simulink model "CryoDetMultiChan_CMB"  (R2016b)
settings: Solver=ode45  StartTime=0.0  StopTime=400e-6  MaxStep=Tclk/4  RelTol=1e-3
values from neighbouring files (symbols this model uses):
  ds_axi = 16    [setupCryoFPGA_CMB.m]
  Fclk = Fadc    (= 307200000)    [setupCryoFPGA_CMB.m]
  lpf = tf(num,den)    [setupCryoFPGA_CMB.m]
  Tclk = 1/Fclk    (= 3.25520833333e-09)    [setupCryoFPGA_CMB.m]
  Ts = 1/Fs    (= 3.25520833333e-09)    [setupADCtoDACloopback.m]    (also in setupCryoFPGA_CMB.m)
undefined symbols (not defined in the file or in its folder): AXI4, i, Lite, xlipgetpartsetting
libraries: xbsIndex_r4 x2215, hdlsllib x6, simulink x3, CryoDetLib x2
(part 5 of 16)

== system CryoDetMultiChan_CMB/DspCore/FTA_Ch0/SixteenLineUDC 0 ==
  note: REF I & Q are in original (unswapped)
      | configuration
  note: SixteenLineUDC(n)
      |
      | Implelents the Up *and* Down Conversion for each Resonator Line/Channel
      | One Block implements one U/D converter pair
      | The counter use used to syncronize the internal CIC filter reset operation to allow the data to be interleaved
      | The MUX16x4 block does the actual time-domain interleaving operation
      | The DC Decimate block does a further decimate and filtering operation on the ADC and Reference signals before sending them downstream for furhter processing
      | The DAC SUM block individually sums the I & Q components of the upconverted signals (4 individual sum streams from the DAC & DAC + phi signals) before they are forwarded downstream.
  ADC_I_in : Inport
  ADC_Q_in : Inport  Port=2
  REF_I_in1 : Inport  Port=3
  REF_Q_in1 : Inport  Port=4
  BDC scope : Scope  NumInputPorts=2
  Constant : xbsIndex_r4/Constant  const=0  gui_display_data_type=Fixed-point  arith_type=Unsigned  n_bits=5  bin_pt=0  preci_type=Single  exp_width=8  frac_width=24  explicit_period=off  period=1  equ=P=C  opselect=C  inp2=PCIN>>17  opr=+  inp1=P  carry=CIN  dbl_ovrd=off  block_type=constant
  Constant1 : xbsIndex_r4/Constant  const=1  gui_display_data_type=Fixed-point  arith_type=Unsigned  n_bits=5  bin_pt=0  preci_type=Single  exp_width=8  frac_width=24  explicit_period=off  period=1  equ=P=C  opselect=C  inp2=PCIN>>17  opr=+  inp1=P  carry=CIN  dbl_ovrd=off  block_type=constant
  Constant10 : xbsIndex_r4/Constant  const=10  gui_display_data_type=Fixed-point  arith_type=Unsigned  n_bits=5  bin_pt=0  preci_type=Single  exp_width=8  frac_width=24  explicit_period=off  period=1  equ=P=C  opselect=C  inp2=PCIN>>17  opr=+  inp1=P  carry=CIN  dbl_ovrd=off  block_type=constant
  Constant11 : xbsIndex_r4/Constant  const=11  gui_display_data_type=Fixed-point  arith_type=Unsigned  n_bits=5  bin_pt=0  preci_type=Single  exp_width=8  frac_width=24  explicit_period=off  period=1  equ=P=C  opselect=C  inp2=PCIN>>17  opr=+  inp1=P  carry=CIN  dbl_ovrd=off  block_type=constant
  Constant12 : xbsIndex_r4/Constant  const=12  gui_display_data_type=Fixed-point  arith_type=Unsigned  n_bits=5  bin_pt=0  preci_type=Single  exp_width=8  frac_width=24  explicit_period=off  period=1  equ=P=C  opselect=C  inp2=PCIN>>17  opr=+  inp1=P  carry=CIN  dbl_ovrd=off  block_type=constant
  Constant13 : xbsIndex_r4/Constant  const=13  gui_display_data_type=Fixed-point  arith_type=Unsigned  n_bits=5  bin_pt=0  preci_type=Single  exp_width=8  frac_width=24  explicit_period=off  period=1  equ=P=C  opselect=C  inp2=PCIN>>17  opr=+  inp1=P  carry=CIN  dbl_ovrd=off  block_type=constant
  Constant14 : xbsIndex_r4/Constant  const=14  gui_display_data_type=Fixed-point  arith_type=Unsigned  n_bits=5  bin_pt=0  preci_type=Single  exp_width=8  frac_width=24  explicit_period=off  period=1  equ=P=C  opselect=C  inp2=PCIN>>17  opr=+  inp1=P  carry=CIN  dbl_ovrd=off  block_type=constant
  Constant15 : xbsIndex_r4/Constant  const=15  gui_display_data_type=Fixed-point  arith_type=Unsigned  n_bits=5  bin_pt=0  preci_type=Single  exp_width=8  frac_width=24  explicit_period=off  period=1  equ=P=C  opselect=C  inp2=PCIN>>17  opr=+  inp1=P  carry=CIN  dbl_ovrd=off  block_type=constant
  Constant2 : xbsIndex_r4/Constant  const=2  gui_display_data_type=Fixed-point  arith_type=Unsigned  n_bits=5  bin_pt=0  preci_type=Single  exp_width=8  frac_width=24  explicit_period=off  period=1  equ=P=C  opselect=C  inp2=PCIN>>17  opr=+  inp1=P  carry=CIN  dbl_ovrd=off  block_type=constant
  Constant20 : xbsIndex_r4/Constant  const=31  gui_display_data_type=Fixed-point  arith_type=Unsigned  n_bits=5  bin_pt=0  preci_type=Single  exp_width=8  frac_width=24  explicit_period=off  period=1  equ=P=C  opselect=C  inp2=PCIN>>17  opr=+  inp1=P  carry=CIN  dbl_ovrd=off  block_type=constant
  Constant3 : xbsIndex_r4/Constant  const=3  gui_display_data_type=Fixed-point  arith_type=Unsigned  n_bits=5  bin_pt=0  preci_type=Single  exp_width=8  frac_width=24  explicit_period=off  period=1  equ=P=C  opselect=C  inp2=PCIN>>17  opr=+  inp1=P  carry=CIN  dbl_ovrd=off  block_type=constant
  Constant4 : xbsIndex_r4/Constant  const=4  gui_display_data_type=Fixed-point  arith_type=Unsigned  n_bits=5  bin_pt=0  preci_type=Single  exp_width=8  frac_width=24  explicit_period=off  period=1  equ=P=C  opselect=C  inp2=PCIN>>17  opr=+  inp1=P  carry=CIN  dbl_ovrd=off  block_type=constant
  Constant5 : xbsIndex_r4/Constant  const=5  gui_display_data_type=Fixed-point  arith_type=Unsigned  n_bits=5  bin_pt=0  preci_type=Single  exp_width=8  frac_width=24  explicit_period=off  period=1  equ=P=C  opselect=C  inp2=PCIN>>17  opr=+  inp1=P  carry=CIN  dbl_ovrd=off  block_type=constant
  Constant6 : xbsIndex_r4/Constant  const=6  gui_display_data_type=Fixed-point  arith_type=Unsigned  n_bits=5  bin_pt=0  preci_type=Single  exp_width=8  frac_width=24  explicit_period=off  period=1  equ=P=C  opselect=C  inp2=PCIN>>17  opr=+  inp1=P  carry=CIN  dbl_ovrd=off  block_type=constant
  Constant7 : xbsIndex_r4/Constant  const=7  gui_display_data_type=Fixed-point  arith_type=Unsigned  n_bits=5  bin_pt=0  preci_type=Single  exp_width=8  frac_width=24  explicit_period=off  period=1  equ=P=C  opselect=C  inp2=PCIN>>17  opr=+  inp1=P  carry=CIN  dbl_ovrd=off  block_type=constant
  Constant8 : xbsIndex_r4/Constant  const=8  gui_display_data_type=Fixed-point  arith_type=Unsigned  n_bits=5  bin_pt=0  preci_type=Single  exp_width=8  frac_width=24  explicit_period=off  period=1  equ=P=C  opselect=C  inp2=PCIN>>17  opr=+  inp1=P  carry=CIN  dbl_ovrd=off  block_type=constant
  Constant9 : xbsIndex_r4/Constant  const=9  gui_display_data_type=Fixed-point  arith_type=Unsigned  n_bits=5  bin_pt=0  preci_type=Single  exp_width=8  frac_width=24  explicit_period=off  period=1  equ=P=C  opselect=C  inp2=PCIN>>17  opr=+  inp1=P  carry=CIN  dbl_ovrd=off  block_type=constant
  Counter : xbsIndex_r4/Counter  cnt_type=Count Limited  cnt_to=31  operation=Up  start_count=0  cnt_by_val=1  arith_type=Unsigned  n_bits=5  bin_pt=0  load_pin=off  rst=on  en=on  explicit_period=off  period=Tclk  use_behavioral_HDL=off  implementation=Fabric  dbl_ovrd=off  block_type=counter
  DAC Sum1 : Subsystem
  DC_decimate : Subsystem
  Delay : xbsIndex_r4/Delay  rst=off  infoeditControl=Selection of Reset will increase slice count due to use of real FFs and instead of SRLs  en=off  latency=6  reg_retiming=off  dbl_ovrd=off  block_type=delay
  Demux : Demux  Outputs=2
  Demux1 : Demux  Outputs=2
  Gateway Out{1,7..10,23} (6 alike) : xbsIndex_r4/Gateway Out  inherit_from_input=off  hdl_port=off  rows=1  columns=1  UseAsDAC=off  DACChannel='1'  interface=None  automatic_assignment=on  address_offset=hex2dec('00')  intf_name=''  intf_description=''  timing_constraint=None  locs_specified=off  LOCs={}  io_standard={}  block_type=gatewayout
  Mux{,1,6..7} (4 alike) : Mux  Inputs=2
  Mux16X4 : Subsystem
  Relational : xbsIndex_r4/Relational  mode=a!=b  op_type=Bool  en=off  latency=0  dbl_ovrd=off  block_type=relational
  debug Scope : Subsystem
  oneLineUpDown0 : Subsystem
  oneLineUpDown1 : Subsystem
  oneLineUpDown10 : Subsystem
  oneLineUpDown11 : Subsystem
  oneLineUpDown12 : Subsystem
  oneLineUpDown13 : Subsystem
  oneLineUpDown14 : Subsystem
  oneLineUpDown15 : Subsystem
  oneLineUpDown2 : Subsystem
  oneLineUpDown3 : Subsystem
  oneLineUpDown4 : Subsystem
  oneLineUpDown5 : Subsystem
  oneLineUpDown6 : Subsystem
  oneLineUpDown7 : Subsystem
  oneLineUpDown8 : Subsystem
  oneLineUpDown9 : Subsystem
  synch scope : Scope  NumInputPorts=2
  toDAC : Outport
  demodulated : Outport  Port=2
  wires:
  [fpgaReset] -> Counter/1, Delay/1
  Gateway Out10/1 -> Mux7/2
  Gateway Out9/1 -> Mux7/1
  Gateway Out8/1 -> Mux6/2
  Gateway Out7/1 -> Mux6/1
  Mux6/1 -> BDC scope/1
  Mux7/1 -> BDC scope/2
  Demux/1 -> Gateway Out7/1
  Demux1/2 -> Gateway Out10/1
  Demux1/1 -> Gateway Out9/1
  Demux/2 -> Gateway Out8/1
  Delay/1 -> Mux16X4/1(synch)
  Constant/1 -> oneLineUpDown0/2(addrIn)
  Counter/1 -> Gateway Out23/1, oneLineUpDown1/3(synchIn), oneLineUpDown2/3(synchIn), oneLineUpDown3/3(synchIn), oneLineUpDown4/3(synchIn), oneLineUpDown5/3(synchIn), oneLineUpDown6/3(synchIn), oneLineUpDown7/3(synchIn), oneLineUpDown8/3(synchIn), oneLineUpDown9/3(synchIn), oneLineUpDown10/3(synchIn), oneLineUpDown11/3(synchIn), oneLineUpDown12/3(synchIn), oneLineUpDown13/3(synchIn), oneLineUpDown15/3(synchIn), oneLineUpDown14/3(synchIn), oneLineUpDown0/3(synchIn), Relational/2
  Gateway Out23/1 -> synch scope/1
  Gateway Out1/1 -> synch scope/2
  Relational/1 -> Gateway Out1/1, Counter/2
  Constant20/1 -> Relational/1
  oneLineUpDown0/1(DC_Out) -> debug Scope/1(demod), Mux16X4/2(line0)  "DC_out_line0"
  oneLineUpDown1/1(DC_Out) -> Mux16X4/3(line1)  "DC_out_line1"
  oneLineUpDown2/1(DC_Out) -> Mux16X4/4(line2)  "DC_out_line2"
  oneLineUpDown3/1(DC_Out) -> Mux16X4/5(line3)  "DC_out_line3"
  oneLineUpDown4/1(DC_Out) -> Mux16X4/6(line4)  "DC_out_line4"
  oneLineUpDown5/1(DC_Out) -> Mux16X4/7(line5)  "DC_out_line5"
  oneLineUpDown6/1(DC_Out) -> Mux16X4/8(line6)  "DC_out_line6"
  oneLineUpDown7/1(DC_Out) -> Mux16X4/9(line7)  "DC_out_line7"
  oneLineUpDown8/1(DC_Out) -> Mux16X4/10(line8)  "DC_out_line8"
  oneLineUpDown9/1(DC_Out) -> Mux16X4/11(line9)  "DC_out_line9"
  oneLineUpDown10/1(DC_Out) -> Mux16X4/12(line10)  "DC_out_line10"
  oneLineUpDown11/1(DC_Out) -> Mux16X4/13(line11)  "DC_out_line11"
  oneLineUpDown12/1(DC_Out) -> Mux16X4/14(line12)  "DC_out_line12"
  oneLineUpDown13/1(DC_Out) -> Mux16X4/15(line13)  "DC_out_line13"
  oneLineUpDown14/1(DC_Out) -> Mux16X4/16(line14)  "DC_out_line14"
  oneLineUpDown15/1(DC_Out) -> Mux16X4/17(line15)  "DC_out_line15"
  oneLineUpDown15/2(UC_out) -> DAC Sum1/1(In1)  "UC_out_line15"
  oneLineUpDown14/2(UC_out) -> DAC Sum1/2(In2)  "UC_out_line14"
  oneLineUpDown13/2(UC_out) -> DAC Sum1/3(In3)  "UC_out_line13"
  oneLineUpDown12/2(UC_out) -> DAC Sum1/4(In4)  "UC_out_line12"
  oneLineUpDown11/2(UC_out) -> DAC Sum1/5(In5)  "UC_out_line11"
  oneLineUpDown10/2(UC_out) -> DAC Sum1/6(In6)  "UC_out_line10"
  oneLineUpDown9/2(UC_out) -> DAC Sum1/7(In7)  "UC_out_line9"
  oneLineUpDown8/2(UC_out) -> DAC Sum1/8(In8)  "UC_out_line8"
  oneLineUpDown7/2(UC_out) -> DAC Sum1/9(In9)  "UC_out_line7"
  oneLineUpDown6/2(UC_out) -> DAC Sum1/10(In10)  "UC_out_line6"
  oneLineUpDown5/2(UC_out) -> DAC Sum1/11(In11)  "UC_out_line5"
  oneLineUpDown4/2(UC_out) -> DAC Sum1/12(In12)  "UC_out_line4"
  oneLineUpDown3/2(UC_out) -> DAC Sum1/13(In13)  "UC_out_line3"
  oneLineUpDown2/2(UC_out) -> DAC Sum1/14(In14)  "UC_out_line2"
  oneLineUpDown1/2(UC_out) -> DAC Sum1/15(In15)  "UC_out_line1"
  oneLineUpDown0/3(UC_out) -> DAC Sum1/16(In16)  "UC_out_line0"
  Constant1/1 -> oneLineUpDown1/2(addrIn)
  Constant2/1 -> oneLineUpDown2/2(addrIn)
  Constant3/1 -> oneLineUpDown3/2(addrIn)
  Constant4/1 -> oneLineUpDown4/2(addrIn)
  Constant5/1 -> oneLineUpDown5/2(addrIn)
  Constant6/1 -> oneLineUpDown6/2(addrIn)
  Constant7/1 -> oneLineUpDown7/2(addrIn)
  Constant8/1 -> oneLineUpDown8/2(addrIn)
  Constant9/1 -> oneLineUpDown9/2(addrIn)
  Constant10/1 -> oneLineUpDown10/2(addrIn)
  Constant11/1 -> oneLineUpDown11/2(addrIn)
  Constant12/1 -> oneLineUpDown12/2(addrIn)
  Constant13/1 -> oneLineUpDown13/2(addrIn)
  Constant14/1 -> oneLineUpDown14/2(addrIn)
  Constant15/1 -> oneLineUpDown15/2(addrIn)
  ADC_Q_in/1 -> Mux/1
  ADC_I_in/1 -> Mux/2
  REF_I_in1/1 -> Mux1/2
  REF_Q_in1/1 -> Mux1/1
  Mux/1 -> oneLineUpDown1/1(ADC_IQ_in), oneLineUpDown2/1(ADC_IQ_in), Demux/1, oneLineUpDown3/1(ADC_IQ_in), oneLineUpDown4/1(ADC_IQ_in), oneLineUpDown5/1(ADC_IQ_in), oneLineUpDown6/1(ADC_IQ_in), oneLineUpDown7/1(ADC_IQ_in), oneLineUpDown8/1(ADC_IQ_in), oneLineUpDown9/1(ADC_IQ_in), oneLineUpDown10/1(ADC_IQ_in), oneLineUpDown11/1(ADC_IQ_in), oneLineUpDown12/1(ADC_IQ_in), oneLineUpDown13/1(ADC_IQ_in), oneLineUpDown15/1(ADC_IQ_in), oneLineUpDown14/1(ADC_IQ_in), oneLineUpDown0/1(ADC_IQ_in)
  Mux1/1 -> oneLineUpDown0/4(REF_IQ_in1), oneLineUpDown1/4(REF_IQ_in1), oneLineUpDown2/4(REF_IQ_in1), oneLineUpDown3/4(REF_IQ_in1), oneLineUpDown4/4(REF_IQ_in1), Demux1/1, oneLineUpDown5/4(REF_IQ_in1), oneLineUpDown6/4(REF_IQ_in1), oneLineUpDown7/4(REF_IQ_in1), oneLineUpDown8/4(REF_IQ_in1), oneLineUpDown9/4(REF_IQ_in1), oneLineUpDown10/4(REF_IQ_in1), oneLineUpDown11/4(REF_IQ_in1), oneLineUpDown12/4(REF_IQ_in1), oneLineUpDown13/4(REF_IQ_in1), oneLineUpDown15/4(REF_IQ_in1), oneLineUpDown14/4(REF_IQ_in1)
  DAC Sum1/1(Out1) -> toDAC/1
  Mux16X4/1(Out1) -> DC_decimate/1(In1)
  DC_decimate/1(dec_sig_ref) -> demodulated/1
  oneLineUpDown0/2(Freq) -> debug Scope/2(freq)

== system CryoDetMultiChan_CMB/DspCore/FTA_Ch0/dF ==
  note: NOTE <11-08-2017 JED>: Connected RE{} output to dFBus now instead of IM{} as was originally
  note: Latency =11
  note: Delay4 + eta mux + cast/covnert total latency = 19
      |
      | Note: this path should match above (multiply) path
  note: Channel
  note: sig0
  note: conj(Ref0)
  note: Match latencies
  note: dF
  note: Ref
  note: Sig
  note: Frequency error dF = Re(eta'*Ref'*Sig)
      | where eta' is like a phase and amplitude calibration including the phase determined by the 2 sidebands and amplitude determined by the reference central line and bandwidth
      |
      | get channel ID
      | fetch eta'
      | calc dF
      | dF now Re{} w/o sidebands <JED: 11-08-2017>
  note: Tvalid
  note: eta mux has latency of 4
  note: Latency =11
  In1 : Inport
  BW : Display
  BW in MHz : Display
  Bus Creator : BusCreator  Inputs=3
  Bus Selector : BusSelector  OutputSignals=chanAndTvalid,decSigandRef
  Bus Selector4 : BusSelector  OutputSignals=Q_Eta,I_Eta
  CMult : xbsIndex_r4/CMult  const=-1  gui_display_data_type=Floating-point  const_n_bits=24  const_bin_pt=22  float_type=Single  exp_bits=8  fraction_bits=24  en=off  latency=3  precision=Full  arith_type="Signed  (2's comp)"  n_bits=24  bin_pt=22  quantization=Truncate  overflow=Wrap  use_behavioral_HDL=on  mem_type=Distributed RAM  pipeline=off  dbl_ovrd=off  block_type=cmult
  Constant : xbsIndex_r4/Constant  const=0  gui_display_data_type=Fixed-point  arith_type=Unsigned  n_bits=4  bin_pt=0  preci_type=Single  exp_width=8  frac_width=24  explicit_period=off  period=1  equ=P=C  opselect=C  inp2=PCIN>>17  opr=+  inp1=P  carry=CIN  dbl_ovrd=off  block_type=constant
  Constant1 : xbsIndex_r4/Constant  const=0  gui_display_data_type=Fixed-point  arith_type=Unsigned  n_bits=4  bin_pt=0  preci_type=Single  exp_width=8  frac_width=24  explicit_period=off  period=1  equ=P=C  opselect=C  inp2=PCIN>>17  opr=+  inp1=P  carry=CIN  dbl_ovrd=off  block_type=constant
  Convert{,1..3,6..7} (6 alike) : xbsIndex_r4/Convert  gui_display_data_type=Floating-point  arith_type=Floating-point  n_bits=16  bin_pt=14  float_type=Single  exp_bits=8  fraction_bits=24  quantization=Truncate  overflow=Wrap  en=off  latency=5  pipeline=off  dbl_ovrd=off  block_type=convert
  Convert10 : xbsIndex_r4/Convert  gui_display_data_type=Fixed-point  arith_type="Signed  (2's comp)"  n_bits=32  bin_pt=30  float_type=Single  exp_bits=8  fraction_bits=24  quantization="Round  (unbiased: +/- Inf)"  overflow=Saturate  en=off  latency=2  pipeline=on  dbl_ovrd=off  block_type=convert
  Convert{8..9,11..13} (5 alike) : xbsIndex_r4/Convert  gui_display_data_type=Fixed-point  arith_type="Signed  (2's comp)"  n_bits=32  bin_pt=30  float_type=Single  exp_bits=8  fraction_bits=24  quantization="Round  (unbiased: +/- Inf)"  overflow=Saturate  en=off  latency=1  pipeline=off  dbl_ovrd=off  block_type=convert
  Convert4 : xbsIndex_r4/Convert  gui_display_data_type=Fixed-point  arith_type="Signed  (2's comp)"  n_bits=32  bin_pt=30  float_type=Single  exp_bits=8  fraction_bits=24  quantization="Round  (unbiased: +/- Inf)"  overflow=Saturate  en=off  latency=2  pipeline=on  dbl_ovrd=off  block_type=convert
  Convert5 : xbsIndex_r4/Convert  gui_display_data_type=Floating-point  arith_type=Floating-point  n_bits=16  bin_pt=14  float_type=Single  exp_bits=8  fraction_bits=24  quantization=Truncate  overflow=Wrap  en=off  latency=4  pipeline=on  dbl_ovrd=off  block_type=convert
  CplxProd : Subsystem
  CplxProd1 : Subsystem
  Delay : xbsIndex_r4/Delay  rst=off  infoeditControl=Selection of Reset will increase slice count due to use of real FFs and instead of SRLs  en=off  latency=3  reg_retiming=on  dbl_ovrd=off  block_type=delay
  Delay1 : xbsIndex_r4/Delay  rst=off  infoeditControl=Selection of Reset will increase slice count due to use of real FFs and instead of SRLs  en=off  latency=3  reg_retiming=on  dbl_ovrd=off  block_type=delay
  Delay2 : xbsIndex_r4/Delay  rst=off  infoeditControl=Selection of Reset will increase slice count due to use of real FFs and instead of SRLs  en=off  latency=3  reg_retiming=on  dbl_ovrd=off  block_type=delay
  Delay3 : xbsIndex_r4/Delay  rst=off  infoeditControl=Selection of Reset will increase slice count due to use of real FFs and instead of SRLs  en=off  latency=36  reg_retiming=on  dbl_ovrd=off  block_type=delay
  Delay4 : xbsIndex_r4/Delay  rst=off  infoeditControl=Selection of Reset will increase slice count due to use of real FFs and instead of SRLs  en=off  latency=10  reg_retiming=on  dbl_ovrd=off  block_type=delay
  Delay5 : xbsIndex_r4/Delay  rst=off  infoeditControl=Selection of Reset will increase slice count due to use of real FFs and instead of SRLs  en=off  latency=8  reg_retiming=on  dbl_ovrd=off  block_type=delay
  Delay6 : xbsIndex_r4/Delay  rst=off  infoeditControl=Selection of Reset will increase slice count due to use of real FFs and instead of SRLs  en=off  latency=6  reg_retiming=on  dbl_ovrd=off  block_type=delay
  Demux{1..4} (4 alike) : Demux  Outputs=2
  Display2 : Display
  Display3 : Display
  Gain : Gain  Gain=307.2
  Gateway Out{1..2,4..10} (9 alike) : xbsIndex_r4/Gateway Out  inherit_from_input=off  hdl_port=off  rows=1  columns=1  UseAsDAC=off  DACChannel='1'  interface=None  automatic_assignment=on  address_offset=hex2dec('00')  intf_name=''  intf_description=''  timing_constraint=None  locs_specified=off  LOCs={}  io_standard={}  block_type=gatewayout
  Gateway Out3 : xbsIndex_r4/Gateway Out  inherit_from_input=on  hdl_port=off  rows=1  columns=1  UseAsDAC=off  DACChannel='1'  interface=None  automatic_assignment=on  address_offset=hex2dec('00')  intf_name=''  intf_description=''  timing_constraint=None  locs_specified=off  LOCs={}  io_standard={}  block_type=gatewayout
  Mult1 : xbsIndex_r4/Mult  precision=Full  arith_type="Signed  (2's comp)"  n_bits=32  bin_pt=30  quantization="Round  (unbiased: +/- Inf)"  overflow=Saturate  en=off  latency=4  use_behavioral_HDL=on  opt=Speed  use_embedded=on  optimum_pipeline=off  pipeline=on  dbl_ovrd=off  use_rpm=on  placement_style=Triangular  block_type=mult
  Mult4 : xbsIndex_r4/Mult  precision=Full  arith_type="Signed  (2's comp)"  n_bits=32  bin_pt=30  quantization="Round  (unbiased: +/- Inf)"  overflow=Saturate  en=off  latency=4  use_behavioral_HDL=on  opt=Speed  use_embedded=on  optimum_pipeline=off  pipeline=on  dbl_ovrd=off  use_rpm=on  placement_style=Triangular  block_type=mult
  Register : xbsIndex_r4/Register  init=0  rst=off  en=on  dbl_ovrd=off  block_type=register
  Register1 : xbsIndex_r4/Register  init=0  rst=off  en=off  dbl_ovrd=off  block_type=register
  Register2 : xbsIndex_r4/Register  init=0  rst=off  en=on  dbl_ovrd=off  block_type=register
  Register8 : xbsIndex_r4/Register  init=0  rst=off  en=off  dbl_ovrd=off  block_type=register
  Relational : xbsIndex_r4/Relational  mode=a=b  op_type=Bool  en=off  latency=0  dbl_ovrd=off  block_type=relational
  Relational1 : xbsIndex_r4/Relational  mode=a=b  op_type=Bool  en=off  latency=0  dbl_ovrd=off  block_type=relational
  dF CplxProd1 scope : Scope  NumInputPorts=8
  dF intermediate : Scope  NumInputPorts=8
  dF output : Scope  NumInputPorts=2
  dF scope1 : Scope  NumInputPorts=3
  eta Mux1 : Subsystem
  Out1 : Outport
  tag scope: REAL_ch0_dF_latched=global, ch0_dF_latched=global, dFbus=global
  wires:
  CMult/1 -> CplxProd/4(Im_B)
  Demux2/1 -> Convert2/1
  Demux2/2 -> Convert3/1
  Delay/1 -> CplxProd/5(Re_B)
  Demux1/2 -> Convert1/1
  Demux1/1 -> Convert/1
  Delay1/1 -> CplxProd/2(Im_A)
  CplxProd1/3(Re_Out) -> Mult1/2, dF CplxProd1 scope/7
  Delay6/1 -> dF intermediate/8, Bus Creator/1  "Dvalid"
  In1/1 -> Bus Selector/1
  Bus Creator/1 -> [dFbus], Out1/1
  Register1/1 -> Convert12/1, Mult1/1, Mult4/1, Gateway Out1/1
  CplxProd1/2(Im_Out) -> Convert11/1, dF CplxProd1 scope/8, Mult4/2
  Demux4/1 -> dF scope1/2, Delay3/1, Delay4/1
  Demux4/2 -> dF scope1/1, Delay5/1
  Bus Selector/1 -> Demux4/1  "<chanAndTvalid>"
  Bus Selector/2 -> dF scope1/3, Demux3/1  "<decSigandRef>"
  Mult4/1 -> Convert13/1, Convert4/1  "freqError"
  Delay3/1 -> Gateway Out6/1, Relational1/1, Relational/1, Gateway Out3/1, Bus Creator/2  "channel"
  Convert3/1 -> Delay/1
  Convert2/1 -> CMult/1
  Convert1/1 -> Delay2/1
  Convert/1 -> Delay1/1
  Delay2/1 -> CplxProd/3(Re_A)
  Delay5/1 -> CplxProd/1(tvalidIn)
  CplxProd/2(Im_Out) -> dF CplxProd1 scope/3, CplxProd1/2(Im_A), Convert8/1
  CplxProd/3(Re_Out) -> dF CplxProd1 scope/2, CplxProd1/3(Re_A), Convert9/1
  Convert6/1 -> dF CplxProd1 scope/5, CplxProd1/4(Im_B)
  Convert7/1 -> dF CplxProd1 scope/4, CplxProd1/5(Re_B)
  CplxProd/1(tvalidOut) -> dF CplxProd1 scope/1, CplxProd1/1(tvalidIn)
  Convert4/1 -> dF intermediate/7, Register/1  "old_freqError"
  Gateway Out4/1 -> [ch0_dF_latched], Display3/1, dF output/2
  Gateway Out3/1 -> dF output/1, Display2/1
  Constant/1 -> Relational/2
  Relational/1 -> Register/2
  Register/1 -> Gateway Out4/1
  [BW] -> Register8/1
  Gateway Out1/1 -> BW/1, Gain/1
  Gain/1 -> BW in MHz/1
  Bus Selector4/1 -> Convert6/1  "<Q_Eta>"
  Bus Selector4/2 -> Convert7/1  "<I_Eta>"
  eta Mux1/1(eta out) -> Bus Selector4/1
  Delay4/1 -> eta Mux1/1(channel)
  Demux3/2 -> Demux2/1
  Demux3/1 -> Demux1/1
  Convert9/1 -> Gateway Out2/1
  Convert8/1 -> Gateway Out5/1
  Convert11/1 -> Gateway Out7/1
  Gateway Out2/1 -> dF intermediate/3
  Gateway Out5/1 -> dF intermediate/2
  Gateway Out6/1 -> dF intermediate/1
  Gateway Out7/1 -> dF intermediate/4
  Convert12/1 -> Gateway Out8/1
  Gateway Out8/1 -> dF intermediate/5
  Convert13/1 -> Gateway Out9/1
  Gateway Out9/1 -> dF intermediate/6
  CplxProd1/1(tvalidOut) -> dF CplxProd1 scope/6, Delay6/1  "Dvalid"
  Register8/1 -> Convert5/1
  Convert5/1 -> Register1/1
  Gateway Out10/1 -> [REAL_ch0_dF_latched]
  Constant1/1 -> Relational1/2
  Relational1/1 -> Register2/2
  Register2/1 -> Gateway Out10/1
  Mult1/1 -> Convert10/1
  Convert10/1 -> Register2/1, Bus Creator/3  "freqError"

== system CryoDetMultiChan_CMB/DspCore/FTA_Ch0/dphi ==
  note: check format of Fbus
  note: scale by 1/2 since phase increment per 1/370 = 1/2 of phase increment per 1/185
  note: dPhi
      | calculate complex phase advance for a single sample of ADC input
      | at the frequency of a single channel and send off on dphiBus
  In1 : Inport
  BitBasher : xbsIndex_r4/BitBasher  bitexpr=a={1'b0, b[23:1]}  display_expr=on  sr_1=a  arith_type1=Unsigned  bin_pt1=24  sr_2=2  arith_type2=Unsigned  bin_pt2=0  sr_3=3  arith_type3=Unsigned  bin_pt3=0  sr_4=4  arith_type4=Unsigned  bin_pt4=0  dbl_ovrd=off  block_type=bitbasher
  Bus Creator : BusCreator  Inputs=3
  Constant : xbsIndex_r4/Constant  const=1  gui_display_data_type=Boolean  arith_type=Boolean  n_bits=16  bin_pt=14  preci_type=Single  exp_width=8  frac_width=24  explicit_period=off  period=1  equ=P=C  opselect=C  inp2=PCIN>>17  opr=+  inp1=P  carry=CIN  dbl_ovrd=off  block_type=constant
  Convert : xbsIndex_r4/Convert  gui_display_data_type=Fixed-point  arith_type=Unsigned  n_bits=16  bin_pt=16  float_type=Single  exp_bits=8  fraction_bits=24  quantization="Round  (unbiased: Even Values)"  overflow=Wrap  en=off  latency=1  pipeline=off  dbl_ovrd=off  block_type=convert
  "DDS Compiler 6.0 " : xbsIndex_r4/DDS Compiler 6.0   partspresent=SIN_COS_LUT_only  dds_clock_rate=100  channels=1  mode_of_operation=Standard  modulus=9  parameter_entry=Hardware_Parameters  spurious_free_dynamic_range=45  frequency_resolution=0.4  noise_shaping=None  phase_width=16  output_width=IQbits  output_selection=Sine_and_Cosine  negative_sine=off  negative_cosine=off  amplitude_mode=Unit_Circle  memory_type=Auto  optimization_goal=Speed  dsp48_use=Maximal  resync=off  latency_configuration=Auto  latency=15  has_phase_out=off  has_aclken=off  has_aresetn=off  explicit_period=on  period=Tclk  data_has_tlast=Not_Required  has_tready=off  s_phase_has_tuser=Not_Required  m_data_has_tuser=Not_Required  m_phase_has_tuser=Not_Required  s_phase_tuser_width=1  output_form=Twos_Complement  s_config_sync_mode=On_Vector  phase_increment=Fixed  output_frequency1=0  output_frequency2=0  output_frequency3=0  output_frequency4=0  output_frequency5=0  output_frequency6=0  output_frequency7=0  output_frequency8=0  output_frequency9=0  output_frequency10=0  output_frequency11=0  output_frequency12=0  output_frequency13=0  output_frequency14=0  output_frequency15=0  output_frequency16=0  pinc1='0'  pinc2='0'  pinc3='0'  pinc4='0'  pinc5='0'  pinc6='0'  pinc7='0'  pinc8='0'  pinc9='0'  pinc10='0'  pinc11='0'  pinc12='0'  pinc13='0'  pinc14='0'  pinc15='0'  pinc16='0'  phase_offset=Programmable  phase_offset_angles1=0  phase_offset_angles2=0  phase_offset_angles3=0  phase_offset_angles4=0  phase_offset_angles5=0  phase_offset_angles6=0  phase_offset_angles7=0  phase_offset_angles8=0  phase_offset_angles9=0  phase_offset_angles10=0  phase_offset_angles11=0  phase_offset_angles12=0  phase_offset_angles13=0  phase_offset_angles14=0  phase_offset_angles15=0  phase_offset_angles16=0  poff1='0'  poff2='0'  poff3='0'  poff4='0'  poff5='0'  poff6='0'  poff7='0'  poff8='0'  poff9='0'  poff10='0'  poff11='0'  poff12='0'  poff13='0'  poff14='0'  poff15='0'  poff16='0'  trim_axipin_name=on  simulation_type=hybrid_sim  simulation_model=sysgen:xddsv6_0_cmodel  data_path_portlist={ 's_axis_config_tdata_poff', 's_axis_config_tdata_chan0_poff', 's_axis_config_tdata_pinc', 's_axis_config_tdata_chan0_pinc', 's_axis_phase_tdata_resync', 's_axis_phase_tdata_chan0_resync', 's_axis_phase_tdata_poff', 's_axis_phase_tdata_chan0_poff', 's_axis_phase_tdata_pinc', 's_axis_phase_tdata_chan0_pinc', 's_axis_phase_tdata_phase_in', 'm_axis_data_tdata_sine', 'm_axis_data_tdata_chan0_sine', 'm_axis_data_tdata_cosine', 'm_axis_data_tdata_chan0_cosine', 'm_axis_phase_tdata_phase_out', 'm_axis_phase_tdata_chan0_phase_out'}  por_mode=false  gui_behaviour=Sysgen  ip_name=DDS Compiler  ip_version=6.0  dsptool_ready=true  wrapper_available=true  port_translation_map={ 'aclken' => 'en', 'aresetn' => 'rst' }  ipcore_usecache=true  ipcore_useipmodelcache=true  ipcore_xco_need_fpga_part=true  ipcore_fpga_part=xlipgetpartsetting(gcb, {'kintex7', 'xc7k325t', '-3', 'fbg676'})  ipcore_verbose=false  block_type=dds_compiler_v6_0
  Delay : xbsIndex_r4/Delay  rst=off  infoeditControl=Selection of Reset will increase slice count due to use of real FFs and instead of SRLs  en=off  latency=7  reg_retiming=off  dbl_ovrd=off  block_type=delay
  Display : Display
  Display1 : Display
  Display2 : Display
  Gateway Out{,1..6} (7 alike) : xbsIndex_r4/Gateway Out  inherit_from_input=off  hdl_port=off  rows=1  columns=1  UseAsDAC=off  DACChannel='1'  interface=None  automatic_assignment=on  address_offset=hex2dec('00')  intf_name=''  intf_description=''  timing_constraint=None  locs_specified=off  LOCs={}  io_standard={}  block_type=gatewayout
  Slice : xbsIndex_r4/Slice  nbits=freqBusAddrBits  boolean_output=off  mode=Lower Bit Location + Width  bit1=0  base1=MSB of Input  bit0=freqBits  base0=LSB of Input  dbl_ovrd=off  block_type=slice
  dphi scope : Scope  NumInputPorts=3
  dphi scope1 : Scope  NumInputPorts=3
  tag scope: dphiBus=scoped
  wires:
  Bus Creator/1 -> [dphiBus]
  BitBasher/1 -> Convert/1, Gateway Out4/1
  Delay/1 -> Bus Creator/1, Gateway Out6/1, Gateway Out2/1  "channel"
  Convert/1 -> Gateway Out5/1, "DDS Compiler 6.0 "/2
  Constant/1 -> "DDS Compiler 6.0 "/1
  "DDS Compiler 6.0 "/2 -> Bus Creator/2, Gateway Out/1  "dPhiQ"
  "DDS Compiler 6.0 "/3 -> Bus Creator/3, Gateway Out1/1  "dPhiI"
  Gateway Out/1 -> dphi scope/2, Display/1
  Gateway Out1/1 -> dphi scope/3, Display1/1
  Gateway Out2/1 -> Display2/1
  In1/1 -> BitBasher/1, Slice/1
  Slice/1 -> Gateway Out3/1, Delay/1
  Gateway Out5/1 -> dphi scope1/3
  Gateway Out4/1 -> dphi scope1/2
  Gateway Out3/1 -> dphi scope1/1
  Gateway Out6/1 -> dphi scope/1

== system CryoDetMultiChan_CMB/DspCore/FTA_Ch0/loopFilter ==
  note: convert to MHz
  note: F out should be Fi + DF
      | where DF is integral of frequency error dF subject to limits and FBen
  note: loopFilter
      | multi-line feedback block
      | mplement intial frequency, limits, integrator, gain
  In1 : Inport
  Assert : xbsIndex_r4/Assert  assert_type=on  type_source=Explicitly  gui_display_data_type=Fixed-point  arith_type=Unsigned  n_bits=5  bin_pt=0  preci_type=Single  exp_width=8  frac_width=24  assert_rate=on  rate_source=Explicitly  period=Tclk  output_port=on  block_type=assert
  Assert1 : xbsIndex_r4/Assert  assert_type=on  type_source=Explicitly  gui_display_data_type=Fixed-point  arith_type="Signed  (2's comp)"  n_bits=32  bin_pt=30  preci_type=Single  exp_width=8  frac_width=24  assert_rate=on  rate_source=Explicitly  period=Tclk  output_port=on  block_type=assert
  Assert2 : xbsIndex_r4/Assert  assert_type=on  type_source=Explicitly  gui_display_data_type=Boolean  arith_type=Boolean  n_bits=16  bin_pt=14  preci_type=Single  exp_width=8  frac_width=24  assert_rate=on  rate_source=Explicitly  period=Tclk  output_port=on  block_type=assert
  Assert3 : xbsIndex_r4/Assert  assert_type=on  type_source=Explicitly  gui_display_data_type=Boolean  arith_type=Boolean  n_bits=16  bin_pt=14  preci_type=Single  exp_width=8  frac_width=24  assert_rate=on  rate_source=Explicitly  period=Tclk  output_port=on  block_type=assert
  Assert4 : xbsIndex_r4/Assert  assert_type=on  type_source=Explicitly  gui_display_data_type=Boolean  arith_type=Boolean  n_bits=16  bin_pt=14  preci_type=Single  exp_width=8  frac_width=24  assert_rate=on  rate_source=Explicitly  period=Tclk  output_port=on  block_type=assert
  Assert5 : xbsIndex_r4/Assert  assert_type=on  type_source=Explicitly  gui_display_data_type=Fixed-point  arith_type=Unsigned  n_bits=25  bin_pt=0  preci_type=Single  exp_width=8  frac_width=24  assert_rate=on  rate_source=Explicitly  period=Tclk  output_port=on  block_type=assert
  Assert6 : xbsIndex_r4/Assert  assert_type=on  type_source=Explicitly  gui_display_data_type=Fixed-point  arith_type=Unsigned  n_bits=16  bin_pt=16  preci_type=Single  exp_width=8  frac_width=24  assert_rate=on  rate_source=Explicitly  period=Tclk  output_port=on  block_type=assert
  Assert8 : xbsIndex_r4/Assert  assert_type=on  type_source=Explicitly  gui_display_data_type=Fixed-point  arith_type=Unsigned  n_bits=24  bin_pt=24  preci_type=Single  exp_width=8  frac_width=24  assert_rate=on  rate_source=Explicitly  period=Tclk  output_port=on  block_type=assert
  Assert9 : xbsIndex_r4/Assert  assert_type=on  type_source=Explicitly  gui_display_data_type=Fixed-point  arith_type=Unsigned  n_bits=5  bin_pt=0  preci_type=Single  exp_width=8  frac_width=24  assert_rate=on  rate_source=Explicitly  period=Tclk  output_port=on  block_type=assert
  Bus Selector : BusSelector  OutputSignals=Dvalid,channel,freqError
  Concat : xbsIndex_r4/Concat  num_inputs=2  dbl_ovrd=off  block_type=concat
  Constant : xbsIndex_r4/Constant  const=0  gui_display_data_type=Fixed-point  arith_type=Unsigned  n_bits=5  bin_pt=0  preci_type=Single  exp_width=8  frac_width=24  explicit_period=off  period=1  equ=P=C  opselect=C  inp2=PCIN>>17  opr=+  inp1=P  carry=CIN  dbl_ovrd=off  block_type=constant
  Constant1 : xbsIndex_r4/Constant  const=0  gui_display_data_type=Fixed-point  arith_type=Unsigned  n_bits=5  bin_pt=0  preci_type=Single  exp_width=8  frac_width=24  explicit_period=off  period=1  equ=P=C  opselect=C  inp2=PCIN>>17  opr=+  inp1=P  carry=CIN  dbl_ovrd=off  block_type=constant
  Constant2 : xbsIndex_r4/Constant  const=1  gui_display_data_type=Fixed-point  arith_type=Unsigned  n_bits=5  bin_pt=0  preci_type=Single  exp_width=8  frac_width=24  explicit_period=off  period=1  equ=P=C  opselect=C  inp2=PCIN>>17  opr=+  inp1=P  carry=CIN  dbl_ovrd=off  block_type=constant
  Delay1 : xbsIndex_r4/Delay  rst=off  infoeditControl=Selection of Reset will increase slice count due to use of real FFs and instead of SRLs  en=off  latency=3  reg_retiming=off  dbl_ovrd=off  block_type=delay
  Delay2 : xbsIndex_r4/Delay  rst=off  infoeditControl=Selection of Reset will increase slice count due to use of real FFs and instead of SRLs  en=off  latency=3  reg_retiming=off  dbl_ovrd=off  block_type=delay
  Delay3 : xbsIndex_r4/Delay  rst=off  infoeditControl=Selection of Reset will increase slice count due to use of real FFs and instead of SRLs  en=off  latency=3  reg_retiming=off  dbl_ovrd=off  block_type=delay
  Display2 : Display
  Display3 : Display
  Display4 : Display
      settings: Format=decimal (Stored Integer)
  Gain1 : Gain  Gain=307.2
  Gain2 : Gain  Gain=307.2
  Gain3 : Gain  Gain=307.2
  Gateway Out{1..4,12} (5 alike) : xbsIndex_r4/Gateway Out  inherit_from_input=off  hdl_port=off  rows=1  columns=1  UseAsDAC=off  DACChannel='1'  interface=None  automatic_assignment=on  address_offset=hex2dec('00')  intf_name=''  intf_description=''  timing_constraint=None  locs_specified=off  LOCs={}  io_standard={}  block_type=gatewayout
  Gateway Out13 : xbsIndex_r4/Gateway Out  inherit_from_input=on  hdl_port=off  rows=1  columns=1  UseAsDAC=off  DACChannel='1'  interface=None  automatic_assignment=on  address_offset=hex2dec('00')  intf_name=''  intf_description=''  timing_constraint=None  locs_specified=off  LOCs={}  io_standard={}  block_type=gatewayout
  Gateway Out5 : xbsIndex_r4/Gateway Out  inherit_from_input=on  hdl_port=off  rows=1  columns=1  UseAsDAC=off  DACChannel='1'  interface=None  automatic_assignment=on  address_offset=hex2dec('00')  intf_name=''  intf_description=''  timing_constraint=None  locs_specified=off  LOCs={}  io_standard={}  block_type=gatewayout
  Logical : xbsIndex_r4/Logical  logical_function=OR  inputs=3  en=off  latency=3  precision=User Defined  arith_type=Boolean  n_bits=1  bin_pt=0  align_bp=on  dbl_ovrd=off  block_type=logical
  MCode : xbsIndex_r4/MCode  mfname=multiLineFeedbackpipelined  explicit_period=on  period=Tclk  inputsTable={'boundInpExpr'=>['','','','','','',''],'inputs'=>['channelNo','deltaF','FBen','Finitial','dFmax','FBclr','Dvalid']}  outputsTable={'outputs'=>['freq','chanOut'],'suppressOut'=>['off','off']}  enable_stdout=off  enable_debug=off  suppress_output=on  defparams={}  hide_port_list={}  dbl_ovrd=off  block_type=mcode
  Mult : xbsIndex_r4/Mult  precision=User Defined  arith_type="Signed  (2's comp)"  n_bits=32  bin_pt=30  quantization=Truncate  overflow=Saturate  en=off  latency=3  use_behavioral_HDL=off  opt=Speed  use_embedded=on  optimum_pipeline=off  pipeline=on  dbl_ovrd=off  use_rpm=on  placement_style=Triangular  block_type=mult
  Mux : xbsIndex_r4/Mux  inputs=2  en=off  latency=1  precision=Full  arith_type=Unsigned  n_bits=16  bin_pt=14  quantization=Truncate  overflow=Wrap  dbl_ovrd=off  block_type=mux
  Negate : xbsIndex_r4/Negate  precision=Full  arith_type=Unsigned  n_bits=16  bin_pt=14  quantization=Truncate  overflow=Wrap  en=off  latency=1  dbl_ovrd=off  block_type=negate
  Register : xbsIndex_r4/Register  init=0  rst=off  en=on  dbl_ovrd=off  block_type=register
  Register1 : xbsIndex_r4/Register  init=0  rst=off  en=on  dbl_ovrd=off  block_type=register
  Register2 : xbsIndex_r4/Register  init=0  rst=off  en=on  dbl_ovrd=off  block_type=register
  Register3 : xbsIndex_r4/Register  init=0  rst=off  en=off  dbl_ovrd=off  block_type=register
  Reinterpret : xbsIndex_r4/Reinterpret  force_arith_type=off  arith_type=Unsigned  force_bin_pt=on  bin_pt=0  block_type=reinterpret
  Relational : xbsIndex_r4/Relational  mode=a=b  op_type=Bool  en=off  latency=0  dbl_ovrd=off  block_type=relational
  Relational1 : xbsIndex_r4/Relational  mode=a=b  op_type=Bool  en=off  latency=0  dbl_ovrd=off  block_type=relational
  Relational2 : xbsIndex_r4/Relational  mode=a=b  op_type=Bool  en=off  latency=0  dbl_ovrd=off  block_type=relational
  initial Frequencies : Subsystem
  loop filter input : Scope  NumInputPorts=5
  loop filter output : Scope  NumInputPorts=3
  loop filter output1 : Scope  NumInputPorts=3
  Out1 : Outport
  tag scope: freqBus=global
  wires:
  In1/1 -> Bus Selector/1
  Bus Selector/2 -> Relational/1, Gateway Out3/1, initial Frequencies/1(channel), Delay3/1  "<channel>"
  Bus Selector/3 -> Gateway Out2/1, Register/1, Mult/1  "<freqError>"
  MCode/2 -> Relational2/2, Relational1/2, Gateway Out12/1, Assert9/1  "channel"
  MCode/1 -> Register2/1, Register1/1, Assert8/1  "frequency"
  Register3/1 -> [freqBus], Out1/1
  [fbPolarity] -> loop filter input/5, Mux/1
  [FBgain] -> Mux/2, Negate/1
  [FBlimit] -> Assert6/1
  initial Frequencies/1(Fi) -> Delay2/1
  Assert/1 -> MCode/1
  Assert1/1 -> MCode/2
  Assert2/1 -> MCode/3
  Assert5/1 -> MCode/4
  Assert6/1 -> MCode/5
  Assert9/1 -> loop filter output1/1, Concat/1
  Assert8/1 -> Reinterpret/1
  Reinterpret/1 -> loop filter output1/2, Concat/2
  Gateway Out13/1 -> Display4/1, Gain1/1
  Gateway Out12/1 -> loop filter output/1
  Gateway Out4/1 -> Gain2/1
  Gateway Out3/1 -> Display2/1, loop filter input/1
  Constant/1 -> Relational/2
  Relational/1 -> Register/2
  Register/1 -> Gateway Out4/1
  Constant1/1 -> Relational1/1
  Relational1/1 -> Register1/2
  Register1/1 -> Gateway Out13/1
  Gain1/1 -> loop filter output/2
  Gain2/1 -> Display3/1, loop filter input/2
  Constant2/1 -> Relational2/1
  Relational2/1 -> Register2/2
  Register2/1 -> Gateway Out5/1
  Gateway Out5/1 -> Gain3/1
  Gain3/1 -> loop filter output/3
  Negate/1 -> Mux/3
  Mult/1 -> Assert1/1
  Mux/1 -> Mult/2
  [fpgaReset] -> Logical/2
  [FBen] -> Logical/1
  Logical/1 -> Assert2/1
  Delay3/1 -> Assert/1
  Delay2/1 -> Assert5/1
  Assert3/1 -> MCode/6
  Assert4/1 -> MCode/7
  Delay1/1 -> Assert4/1
  Bus Selector/1 -> Delay1/1, Gateway Out1/1  "<Dvalid>"
  [FBreset] -> Logical/3, Assert3/1
  Concat/1 -> Register3/1
  Gateway Out1/1 -> loop filter input/3
  Gateway Out2/1 -> loop filter input/4
